simulink library "INT_TSDa_tClnt"  (R2016b)
settings: Solver=VariableStepAuto  StartTime=0.0  StopTime=10.0  RelTol=1e-3
settings Model: Creator=xinchangran  LastModifiedBy=xinchangran

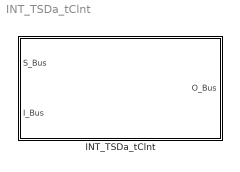
== system INT_TSDa_tClnt ==
  INT_TSDa_tClnt : Subsystem

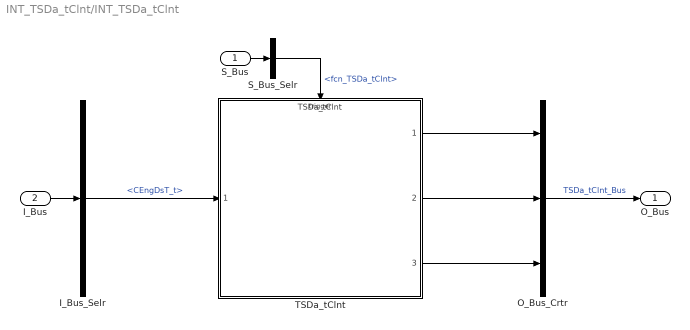
== system INT_TSDa_tClnt/INT_TSDa_tClnt ==
  S_Bus : Inport
  I_Bus : Inport  Port=2
  I_Bus_Selr : BusSelector  OutputSignals=CEngDsT_t
  O_Bus_Crtr : BusCreator  Inputs=3
  S_Bus_Selr : BusSelector  OutputSignals=fcn_TSDa_tClnt
  TSDa_tClnt : ModelReference  ModelNameDialog=TSDa_tClnt  SimulationMode=Normal  ModelReferenceVersion=1.11  TriggerPortName=function  TriggerPortTriggerType=function-call  TriggerPortStatesWhenEnabling=held
  O_Bus : Outport
  wires:
  S_Bus_Selr/1 -> TSDa_tClnt/Trigger  "<fcn_TSDa_tClnt>"
  S_Bus/1 -> S_Bus_Selr/1
  I_Bus/1 -> I_Bus_Selr/1
  I_Bus_Selr/1 -> TSDa_tClnt/1  "<CEngDsT_t>"
  O_Bus_Crtr/1 -> O_Bus/1  "TSDa_tClnt_Bus"
  TSDa_tClnt/1 -> O_Bus_Crtr/1
  TSDa_tClnt/2 -> O_Bus_Crtr/2
  TSDa_tClnt/3 -> O_Bus_Crtr/3
